simulink model "Simulink_EI"  (R2024b)
settings: Solver=ode23tb  StartTime=0.0  StopTime=20  FixedStep=0.00694  RelTol=1e-3
values from neighbouring files (symbols this model uses):
  beta = 1/1820.89    (= 0.000549181993421)    [Matlab_EI_1.m]
  Hco2 = 4003    [Matlab_EI_1.m]
  Ho2 = 94565    [Matlab_EI_1.m]
  phi = 0.2029    [Matlab_EI_1.m]
libraries: slpidlib x6
(part 2 of 2)

== matlab function Simulink_EI/Blé3/MATLAB Function3 ==
  data: Gc input; P_O2_b input; P_CO2_b input; P_O2_c input; P_CO2_c input; dx output
function dx = ble(Gc,P_O2_b,P_CO2_b,P_O2_c,P_CO2_c)

%Gc = 13680;
R  = 8.314;    % [J/(mol·K)]
Tb  = 296;      % [K] 
S = 44.98;
phi = 0.2029;
Vb = S;
T_ref = 298;

H = 20;            % Durée d'ensoleillement en heures (à définir)
C = 0.68;          % Coefficient d'efficacité (à définir)
A_max = 0.93;        % Surface maximale (à définir)
F = 1.4*10^(-3)*24*3600;            % Facteur de flux (à définir)
t_q = 33;          % Durée de photosynthèse active (à définir)
t_a = 12;      % Temps de démarrage de la photosynthèse (à définir)
t_m = 62;          % Durée totale de mesure (à définir)

q_max = 0.05 + 1.437e-4 * (P_CO2_b - 33);
q_min = 0.01 + 2.87e-5 * (P_CO2_b - 33);
P_g = 0.5 * A_max * F * (q_max * (1 + (t_q - t_a) / t_m) + q_min * (1 - t_q / t_m));

dx = zeros(2,1);

P_24_j = (H*C*P_g/24) + (1-C)*4*P_g/24;

k1 = (1-phi)*Gc*Tb / (Vb*T_ref);
k2 = P_24_j*R*Tb*S / Vb;

dx(1) = k1 * (P_O2_c - P_O2_b) + k2 ;   
dx(2) = k1 * (P_CO2_c - P_CO2_b) - k2;

== matlab function Simulink_EI/Habitacle4/MATLAB Function3 ==
  data: Gc input; P_O2_c input; P_CO2_c input; dx output; P_O2_e input; P_CO2_e input; dotOmega_O2 input; dotOmega_CO2 input
function dx = Habitacle(Gc,P_O2_c,P_CO2_c,P_O2_e,P_CO2_e,dotOmega_O2,dotOmega_CO2)

%Gc = 13680;     
Vc = 125;    % [m³]
R  = 8.314;    % [J/(mol·K)]
Tc  = 296;      % [K]
Np = 5;      
%dotOmega_O2 = -1.065*24;
%dotOmega_CO2 =  0.982*24;
T_ref = 298;

dx = zeros(2,1);

k1 = Gc*Tc / (Vc*T_ref);
k2 = R * Tc * Np / Vc;

dx(1) = k1 * (P_O2_e - P_O2_c) + k2 * dotOmega_O2;   % dP_O2^c / dt
dx(2) = k1 * (P_CO2_e - P_CO2_c) + k2 * dotOmega_CO2;   % dP_CO2^c / dt

== matlab function Simulink_EI/Habitacle/MATLAB Function ==
  data: P_O2_c input; P_CO2_c input; dx output; P_O2_e input; P_CO2_e input
function dx = Habitacle(P_O2_c,P_CO2_c,P_O2_e,P_CO2_e)

Gc = 13680;     
Vc = 125;    % [m³]
R  = 8.314;    % [J/(mol·K)]
T  = 298;      % [K]
Np = 5;      
dotOmega_O2 = -0.818;
dotOmega_CO2 =  1.037;

dx = zeros(2,1);

k1 = Gc / Vc;
k2 = R * T * Np / Vc;

dx(1) = k1 * (P_O2_e - P_O2_c) + k2 * dotOmega_O2;   % dP_O2^c / dt
dx(2) = k1 * (P_CO2_e - P_CO2_c) + k2 * dotOmega_CO2;   % dP_CO2^c / dt

== matlab function Simulink_EI/MATLAB Function ==
  data: P_O2_c input; P_CO2_c input; dx output; P_O2_e input; P_CO2_e input
function dx = Habitacle(P_O2_c,P_CO2_c,P_O2_e,P_CO2_e)

Gc = 13680;     
Vc = 125;    % [m³]
R  = 8.314;    % [J/(mol·K)]
Tc  = 296;      % [K]
Np = 5;      
dotOmega_O2 = -1.065*24;
dotOmega_CO2 =  0.982*24;
T_ref = 298;

dx = zeros(2,1);

k1 = Gc*Tc / (Vc*T_ref);
k2 = R * Tc * Np / Vc;

dx(1) = k1 * (P_O2_e - P_O2_c) + k2 * dotOmega_O2;   % dP_O2^c / dt
dx(2) = k1 * (P_CO2_e - P_CO2_c) + k2 * dotOmega_CO2;   % dP_CO2^c / dt

== matlab function Simulink_EI/MATLAB Function1 ==
  data: Cx input; C_O2 input; C_CO2_CT input; P_O2_c input; P_CO2_c input; dx output
function dx = algue(Cx,C_O2,C_CO2_CT,P_O2_c,P_CO2_c)

Gc = 13680;
R  = 8.314;    % [J/(mol·K)]
Vl = 0.384;
phi = 0.2029;
Qp = 1.4285;
H_O2 = 94565;
H_CO2 = 4003;
Mx = 0.0241;
beta = 1/1820.89;
phi0 = 350;
L = 0.018;
m = 310;
mu_M = 0.143*24;
KJ = 40;
T_ref = 298;

Lr = 0.52992;

L2 = log(phi0) / (m * Cx);
Lmin = min(L2, L);
rx = (mu_M / (m*L)) * log( (phi0 + KJ) / (phi0 * exp(-m * Cx * Lmin) + KJ) );

dx = zeros(3,1);

k1 = phi*Gc / (Vl*R*T_ref);
k2 = rx/Mx;

dx(1) = k1 * (P_O2_c - H_O2*C_O2) + k2 * Qp;   
dx(2) = k1 * (P_CO2_c - H_CO2*C_CO2_CT*beta) - k2;  
dx(3) = rx - Lr*Cx/Vl;

== matlab function Simulink_EI/C-IV a : algue/MATLAB Function1 ==
  data: P_O2_a input; P_CO2_a input; P_O2_c input; P_CO2_c input; dx output
function dx = algue(P_O2_a,P_CO2_a,P_O2_c,P_CO2_c)

Gc = 13680;
R  = 8.314;    % [J/(mol·K)]
T  = 309;      % [K] 
Vl = 0.384;
phi = 0.2029;
rx = 1.38;
Qp = 1.4285;
H_O2 = 94565;
H_CO2 = 4003;
Mx = 0.0241;
beta = 1820.89;

dx = zeros(2,1);

k1 = phi*Gc / Vl;
k2 = rx*R*T/Mx;

dx(1) = k1 * (P_O2_c - H_O2*R*T*P_O2_a/beta) + k2 * Qp;   
dx(2) = k1 * (P_CO2_c - H_CO2*R*T*P_CO2_a/beta) + k2;

== matlab function Simulink_EI/MATLAB Function2 ==
  data: P_O2_b input; P_CO2_b input; P_O2_c input; P_CO2_c input; dx output
function dx = ble(P_O2_b,P_CO2_b,P_O2_c,P_CO2_c)

Gc = 13680;
R  = 8.314;    % [J/(mol·K)]
Tb  = 296;      % [K] 
S = 44.98;
phi = 0.2029;
Vb = S;
T_ref = 298;

H = 20;            % Durée d'ensoleillement en heures (à définir)
C = 0.68;          % Coefficient d'efficacité (à définir)
A_max = 0.93;        % Surface maximale (à définir)
F = 1.4*10^(-3)*24*3600;            % Facteur de flux (à définir)
t_q = 33;          % Durée de photosynthèse active (à définir)
t_a = 12;      % Temps de démarrage de la photosynthèse (à définir)
t_m = 62;          % Durée totale de mesure (à définir)

q_max = 0.05 + 1.437e-4 * (P_CO2_b - 33);
q_min = 0.01 + 2.87e-5 * (P_CO2_b - 33);
P_g = 0.5 * A_max * F * (q_max * (1 + (t_q - t_a) / t_m) + q_min * (1 - t_q / t_m));

dx = zeros(2,1);

P_24_j = (H*C*P_g/24) + (1-C)*4*P_g/24;

k1 = (1-phi)*Gc*Tb / (Vb*T_ref);
k2 = P_24_j*R*Tb*S / Vb;

dx(1) = k1 * (P_O2_c - P_O2_b) + k2 ;   
dx(2) = k1 * (P_CO2_c - P_CO2_b) - k2;

== matlab function Simulink_EI/C-IV b : blé/MATLAB Function2 ==
  data: P_O2_b input; P_CO2_b input; P_O2_c input; P_CO2_c input; dx output
function dx = ble(P_O2_b,P_CO2_b,P_O2_c,P_CO2_c)

Gc = 13680;
R  = 8.314;    % [J/(mol·K)]
T  = 296;      % [K] 
S = 44.98;
phi = 0.2029;
Vb = S;
P_24_j = 2.084;

dx = zeros(2,1);

k1 = (1-phi)*Gc / Vb;
k2 = P_24_j*R*T*S / Vb;

dx(1) = k1 * (P_O2_c - P_O2_b) + k2 ;   
dx(2) = k1 * (P_CO2_c - P_CO2_b) - k2;

== matlab function Simulink_EI/Habitacle1/MATLAB Function3 ==
  data: P_O2_c input; P_CO2_c input; dx output; P_O2_e input; P_CO2_e input
function dx = Habitacle(P_O2_c,P_CO2_c,P_O2_e,P_CO2_e)

Gc = 13680;     
Vc = 125;    % [m³]
R  = 8.314;    % [J/(mol·K)]
Tc  = 296;      % [K]
Np = 5;      
dotOmega_O2 = -1.065*24;
dotOmega_CO2 =  0.982*24;
T_ref = 298;

dx = zeros(2,1);

k1 = Gc*Tc / (Vc*T_ref);
k2 = R * Tc * Np / Vc;

dx(1) = k1 * (P_O2_e - P_O2_c) + k2 * dotOmega_O2;   % dP_O2^c / dt
dx(2) = k1 * (P_CO2_e - P_CO2_c) + k2 * dotOmega_CO2;   % dP_CO2^c / dt

== matlab function Simulink_EI/Algue/MATLAB Function3 ==
  data: Cx input; C_O2 input; C_CO2_CT input; P_O2_c input; P_CO2_c input; dx output
function dx = algue(Cx,C_O2,C_CO2_CT,P_O2_c,P_CO2_c)

Gc = 13680;
R  = 8.314;    % [J/(mol·K)]
Vl = 0.384;
phi = 0.2029;
Qp = 1.4285;
H_O2 = 94565;
H_CO2 = 4003;
Mx = 0.0222;
beta = 1/1820.89;
phi0 = 350;
L = 0.018;
m = 310;
mu_M = 0.143*24;
KJ = 40;
T_ref = 298;

Lr = 0.52992;

L2 = log(phi0) / (m * Cx);
Lmin = min(L2, L);
rx = (mu_M / (m*L)) * log( (phi0 + KJ) / (phi0 * exp(-m * Cx * Lmin) + KJ) );

dx = zeros(3,1);

k1 = phi*Gc / (Vl*R*T_ref);
k2 = rx/Mx;

dx(1) = k1 * (P_O2_c - H_O2*C_O2) + k2 * Qp;   
dx(2) = k1 * (P_CO2_c - H_CO2*C_CO2_CT*beta) - k2;  
dx(3) = rx - Lr*Cx/Vl;
